simulink model "static_arc_test"  (R2025b)
settings: Solver=VariableStepAuto  StartTime=0.0  StopTime=10  RelTol=1e-3
libraries: eeRmsMeasurement x1, simulink x1
settings Model: Creator=LYG  LastModifiedBy=LYG

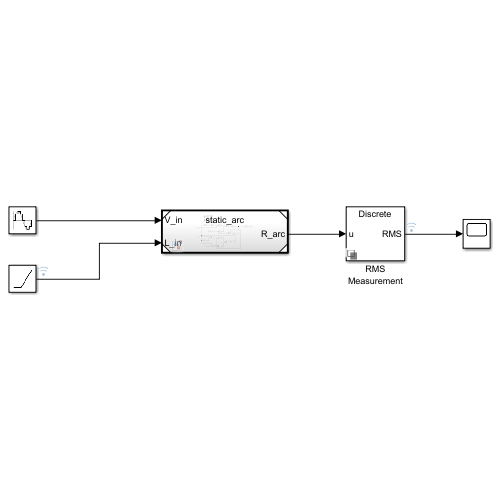
[thumbnail: Simulink's stored preview of the top-level diagram]
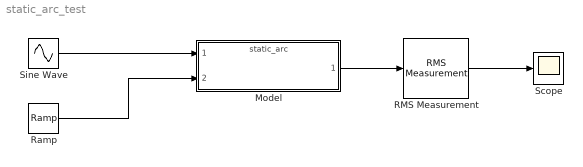
== system static_arc_test ==
  Model : ModelReference  ModelNameDialog=static_arc.slx  SimulationMode=Normal  ModelReferenceVersion=1.7
  RMS Measurement : eeRmsMeasurement/RMS Measurement  LabelModeActiveChoice=Total  F=50  SpecifyHarmonics=off  K=[0 1 2]  Ts=1e-5
      settings: LibrarySourceBlock=|
      | ee_sl_lib/Measurements/RMS
      | Measurement
  Ramp : simulink/Sources/Ramp  slope=(0.7 - 0.1) / 10  start=0  InitialOutput=0.1
  Scope : Scope
      settings: ActiveDisplayYMinimum=-0.0002034056521694437  ActiveDisplayYMaximum=0.016839020680203848
  Sine Wave : Sin  Amplitude=sqrt(2) * 650  Frequency=2 * pi * 50  SampleTime=1e-5
  wires:
  Sine Wave/1 -> Model/1
  Model/1 -> RMS Measurement/1
  RMS Measurement/1 -> Scope/1
  Ramp/1 -> Model/2
